simulink model "cosimulation"  (R2025b)
settings: Solver=FixedStepAuto  StartTime=0.0  StopTime=11  RelTol=1e-3
undefined symbols (not defined in the file or in its folder): gray
libraries: fillib x3, visionsources x1
settings Model: Creator=llillo  LastModifiedBy=llillo
settings OptimizationCC: BlockReduction=off  DefaultParameterBehavior=Inlined  OptimizeBlockIOStorage=off  EnhancedBackFolding=on  PassReuseOutputArgsAs=Individual arguments  OptimizeBlockOrder=speed  DifferentSizesBufferReuse=on  EfficientTunableParamExpr=on
settings DebuggingCC: ParameterTunabilityLossMsg=error
settings HardwareCC: TargetBitPerPointer=64.0  TargetBitPerSizeT=64.0  TargetBitPerPtrDiffT=64.0  TargetLongLongMode=on  TargetIntDivRoundTo=Zero  TargetEndianess=LittleEndian  TargetWordSize=64.0  TargetHWDeviceType=Generic->Custom  ProdEqTarget=off
settings SFSimCC: MATLABDynamicMemAlloc=off
settings RTWCC: SystemTargetFile=systemverilog_dpi_ert.tlc  TemplateMakefile=systemverilog_dpi_ert_default_tmf  Description=SystemVerilog DPI Component Generator
settings CodeAppCC: ForceParamTrailComments=on  IgnoreCustomStorageClasses=off  MaxIdLength=256.0  OperatorAnnotations=on  SimulinkDataObjDesc=on  SFDataObjDesc=on  InsertBlockDesc=on
settings DPIERTTargetCC: DPICustomizeSystemVerilogCode=off  DPISystemVerilogTemplate=svdpi_event.vgt  DPIReportRunTimeError=off  DPIScalarizePorts=off  DPIRunTimeErrorSeverity=Fatal  DPIGenerateTestBench=off  DPIFloatingPointTolerance=4.4409e-16  DPITestBenchSimulator=Siemens Questa/ModelSim  DPITestPointAccessFcnInterface=None  DPIFixedPointDataType=CompatibleCType  DPIPortConnection=Port list  DPICompositeDataType=Flattened  DPIComponentTemplateType=Sequential  DSAsUniqueAccess=off  ExtMode=off  ExtModeTransport=0.0  ExtModeStaticAlloc=off  ExtModeAutomaticAllocSize=on  ExtModeMaxTrigDuration=10.0  ExtModeStaticAllocSize=1000000.0  ExtModeTesting=off  ExtModeMexFile=ext_comm  ExtModeIntrfLevel=Level1  InlinedParameterPlacement=NonHierarchical  TargetOS=BareBoardExample  MultiInstanceErrorCode=Error  RootIOFormat=Part of model data structure  SubcomponentRootIOFormat=Auto  RTWCAPISignals=on  RTWCAPIParams=off  RTWCAPIStates=off  RTWCAPIRootIO=off  ERTSrcFileBannerTemplate=ert_code_template.cgt  ERTHdrFileBannerTemplate=ert_code_template.cgt  ERTDataSrcFileTemplate=ert_code_template.cgt  ERTDataHdrFileTemplate=ert_code_template.cgt  ERTCustomFileTemplate=example_file_process.tlc  EnableDataOwnership=off  SignalDisplayLevel=10.0  ParamTuneLevel=10.0  GlobalDataDefinition=Auto  DataDefinitionFile=global.c  GlobalDataReference=Auto  ERTFilePackagingFormat=Modular  RateTransitionBlockCode=Inline  DataReferenceFile=global.h  PreserveExpressionOrder=off  PreserveIfCondition=off  ConvertIfToSwitch=on  PreserveExternInFcnDecls=on  PreserveStaticInFcnDecls=on  SuppressUnreachableDefaultCases=on  EnableSignedLeftShifts=on  EnableSignedRightShifts=on  ImplementImageWithCVMat=off  IndentStyle=K&R  IndentSize=2  NewlineStyle=Default  MaxLineWidth=80.0  EnableUserReplacementTypes=off  MaxIdInt64=MAX_int64_T  MinIdInt64=MIN_int64_T  MaxIdUint64=MAX_uint64_T  MaxIdInt32=MAX_int32_T  MinIdInt32=MIN_int32_T  MaxIdUint32=MAX_uint32_T  MaxIdInt16=MAX_int16_T  MinIdInt16=MIN_int16_T  MaxIdUint16=MAX_uint16_T  MaxIdInt8=MAX_int8_T  MinIdInt8=MIN_int8_T  MaxIdUint8=MAX_uint8_T  BooleanTrueId=true  BooleanFalseId=false  MemSecPackage=--- None ---  MemSecDataConstants=Default  MemSecDataIO=Default  MemSecDataInternal=Default  MemSecDataParameters=Default  MemSecFuncInitTerm=Default  MemSecFuncExecute=Default  MemSecFuncSharedUtil=Default  GroupConstants=Default  GroupRootInputs=Default  GroupRootOutputs=Default  GroupInternal=Default  GroupParameters=Default  GroupDataTransfer=Default  GroupSharedLocalDataStores=Default  GroupInstanceSpecificParameters=Default  GroupModelData=Default  ArrayContainerType=C-style array  DynamicArrayContainerType=std::vector  TargetFcnLib=ansi_tfl_table_tmw.mat  GenFloatMathFcnCalls=NOT IN USE  TargetLangStandard=C99 (ISO)  CodeReplacementLibrary=None  UtilityFuncGeneration=Auto  MultiwordTypeDef=System defined  MultiwordLength=2048.0  DynamicStringBufferSize=256.0  GenerateFullHeader=on  InferredTypesCompatibility=off  GenerateSampleERTMain=off  GenerateTestInterfaces=off  ModelReferenceCompliant=on  ParMdlRefBuildCompliant=on  CompOptLevelCompliant=on  ConcurrentExecutionCompliant=off  IncludeMdlTerminateFcn=on  CombineOutputUpdateFcns=off  CombineSignalStateStructs=on  GroupInternalDataByFunction=off  SuppressErrorStatus=off  IncludeFileDelimiter=Auto  ERTCustomFileBanners=on  SupportAbsoluteTime=on  LogVarNameModifier=rt_  MatFileLogging=off  PreserveMATLABNamespacesInGeneratedCode=on  CodeInterfacePackaging=Reusable function  SubcomponentCodeInterfacePackaging=Reusable function  PurelyIntegerCode=off  SupportNonFinite=on  SupportComplex=on  SupportContinuousTime=on  SupportNonInlinedSFcns=on  RemoveDisableFunc=off  RemoveResetFunc=on  SupportVariableSizeSignals=off  ParenthesesLevel=Nominal  CastingMode=Nominal  MATLABClassNameForMDSCustomization=Simulink.SoftwareTarget.TargetSpecificTriggerConfigurationBase  ModelStepFunctionPrototypeControlCompliant=on  CPPClassGenCompliant=off  AutosarCompliant=off  MDXCompliant=off  GRTInterface=off  GenerateAllocFcn=on  UseToolchainInfoCompliant=on  GenerateSharedConstants=on  CoderGroups=[]  AccessMethods=[]  LookupTableObjectStructAxisOrder=1,2,3,4,...  LUTObjectStructOrderExplicitValues=Size,Breakpoints,Table  LUTObjectStructOrderEvenSpacing=Size,Breakpoints,Table  ArrayLayout=Column-major  UnsupportedSFcnMsg=error  ERTHeaderFileRootName=$R$E  ERTSourceFileRootName=$R$E  ERTDataFileRootName=$R_data  InstructionSetFMA=off  OptimizeReductions=off  LogToMDFFile=off

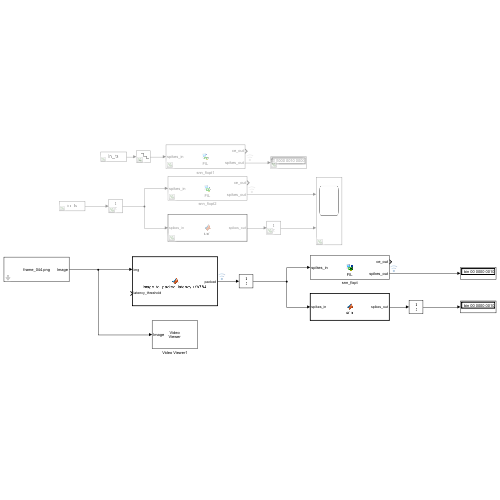
[thumbnail: Simulink's stored preview of the top-level diagram]
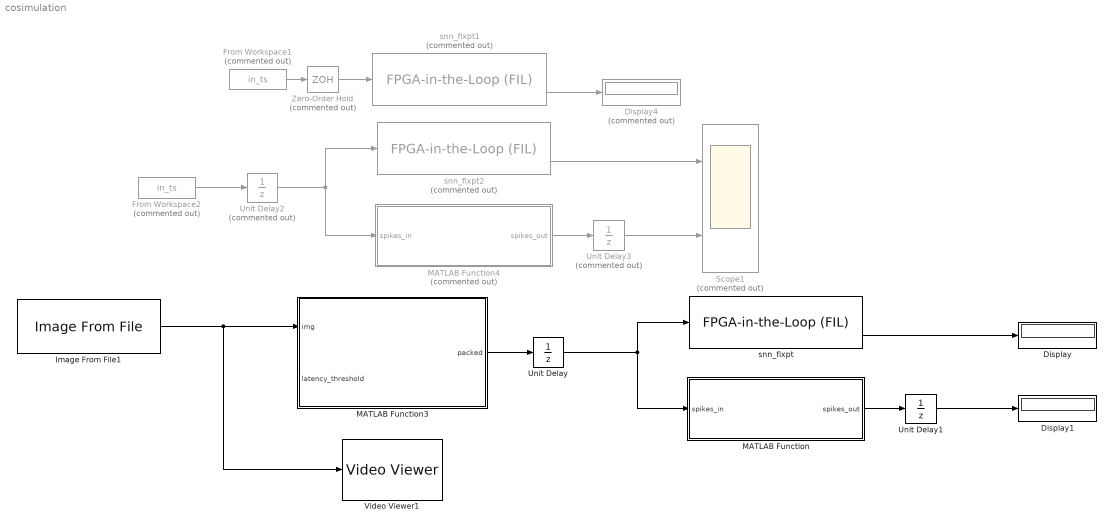
== system cosimulation ==
  Display : Display
      settings: Format=binary (Stored Integer)
  Display1 : Display
      settings: Format=binary (Stored Integer)
  Display4 : Display  Commented=on
      settings: Format=binary (Stored Integer)
  From Workspace1 : FromWorkspace  Commented=on  VariableName=in_ts  SampleTime=0.1  Interpolate=off  OutputAfterFinalValue=Holding final value
  From Workspace2 : FromWorkspace  Commented=on  VariableName=in_ts  SampleTime=0.1  Interpolate=off  OutputAfterFinalValue=Holding final value
  Image From File1 : visionsources/Image From File  Tag=vipblks_nd  FileName=C:\Users\llillo\Desktop\cosas_ordenadas\uni\memoria\git\memoria_fpga_design_matlab\examples\snn_matlab\frames\frame_044.png  Ts=inf  imagePorts=One multidimensional signal  OutPortLabels=R|G|B  ImageDataType=double  sdImageDataType=uint(8)  Signed=on  WordLength=16  FractionLengthMode=User-defined  FractionLength=15
  MATLAB Function : MATLAB Function  TreatAsAtomicUnit=on
  MATLAB Function3 : MATLAB Function  TreatAsAtomicUnit=on
  MATLAB Function4 : MATLAB Function  Commented=on  TreatAsAtomicUnit=on
  Scope1 : Scope  Commented=on  NumInputPorts=2
      settings: ActiveDisplayYMinimum=-64.249999999999986  ActiveDisplayYMaximum=578.25
  Unit Delay : UnitDelay  SampleTime=0.1  HasFrameUpgradeWarning=on
  Unit Delay1 : UnitDelay  SampleTime=0.1  HasFrameUpgradeWarning=on
  Unit Delay2 : UnitDelay  Commented=on  SampleTime=0.1  HasFrameUpgradeWarning=on
  Unit Delay3 : UnitDelay  Commented=on  SampleTime=0.1  HasFrameUpgradeWarning=on
  Video Viewer1 : VideoViewer  colormapValue=gray(256)  FigPos=[1062 715 208 67]
  Zero-Order Hold : ZeroOrderHold  Commented=on  SampleTime=0.1
  snn_fixpt : fillib/FPGA-in-the-Loop (FIL)  ForceInterfaceUpdate=0.90579
  snn_fixpt1 : fillib/FPGA-in-the-Loop (FIL)  Commented=on  ForceInterfaceUpdate=0.81472
  snn_fixpt2 : fillib/FPGA-in-the-Loop (FIL)  Commented=on  ForceInterfaceUpdate=0.90579
  wires:
  Unit Delay/1 -> MATLAB Function/1(spikes_in), snn_fixpt/1
  MATLAB Function/1(spikes_out) -> Unit Delay1/1
  From Workspace1/1 -> Zero-Order Hold/1
  snn_fixpt1/2 -> Display4/1
  Zero-Order Hold/1 -> snn_fixpt1/1
  Unit Delay1/1 -> Display1/1
  snn_fixpt/2 -> Display/1
  From Workspace2/1 -> Unit Delay2/1
  Unit Delay3/1 -> Scope1/2
  MATLAB Function4/1(spikes_out) -> Unit Delay3/1
  snn_fixpt2/2 -> Scope1/1
  Unit Delay2/1 -> snn_fixpt2/1, MATLAB Function4/1(spikes_in)
  MATLAB Function3/1(packed) -> Unit Delay/1
  Image From File1/1 -> Video Viewer1/1, MATLAB Function3/1(img)

== matlab function cosimulation/MATLAB Function ==
  data: spikes_in input; spikes_out output
function spikes_out = snn(spikes_in)
    params = snn_params();
    W = params.W;
    thresh = 1;

    [M, N] = size(W);        % M=784, N=10

    spikes_out = fi(0, 0, N, 0);  % ufix10

    for j = 1:N
        acc = 0;
        for i = 1:M
            % OJO: define el mapeo de bits.
            % Aquí asumo bit 1 = LSB, y que i=1 corresponde al MSB:
            if bitget(spikes_in, M - i + 1)
                acc = acc + W(i,j);
            end
        end

        if acc >= thresh
            % j=1 como MSB de la salida (consistente con lo de arriba)
            spikes_out = bitset(spikes_out, N - j + 1, 1);
        end
    end
end

== matlab function cosimulation/MATLAB Function4 ==
  data: spikes_in input; spikes_out output
function spikes_out = snn(spikes_in)
    params = snn_params();
    W = params.W;
    thresh = 1;

    [M, N] = size(W);        % M=784, N=10

    spikes_out = fi(0, 0, N, 0);  % ufix10

    for j = 1:N
        acc = 0;
        for i = 1:M
            % OJO: define el mapeo de bits.
            % Aquí asumo bit 1 = LSB, y que i=1 corresponde al MSB:
            if bitget(spikes_in, M - i + 1)
                acc = acc + W(i,j);
            end
        end

        if acc >= thresh
            % j=1 como MSB de la salida (consistente con lo de arriba)
            spikes_out = bitset(spikes_out, N - j + 1, 1);
        end
    end
end

== matlab function cosimulation/MATLAB Function3 ==
  data: img input; packed output; latency_threshold input
function packed = image_to_packed_latency_ufix784(img, latency_threshold)

    if nargin < 2 || isempty(latency_threshold)
        latency_threshold = 0.5;
    end

    if ~isa(img, 'double')
        img = double(img);
    end

    if ndims(img) == 3
        if ~isequal(size(img), [28 28 3])
            error('La imagen debe ser 28x28x3.');
        end
        img_gray = rgb2gray(img / max(255, max(img(:))));
    else
        if ~isequal(size(img), [28 28])
            error('La imagen debe ser 28x28.');
        end
        img_gray = img / max(255, max(img(:)));
    end

    spikes = (img_gray.' > latency_threshold);

    packed = fi(0, 0, 784, 0);
    for i = 1:784
        packed = bitset(packed, 784 - i + 1, spikes(i));
    end
end
